simulink model "qpsk_tx"  (R2018a)
settings: Solver=VariableStepAuto  StartTime=0.0  StopTime=1e-6  RelTol=1e-3
libraries: simulink x2, commdigbbndpm3 x1, commfilt2 x1
settings Model: Creator=alist  LastModifiedBy=alist

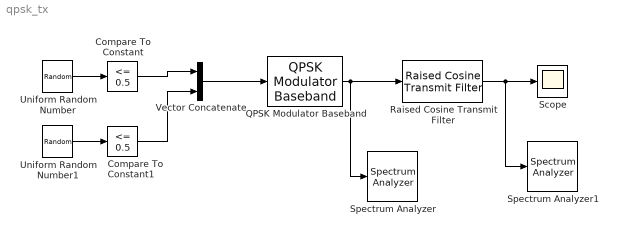
== system qpsk_tx ==
  Compare To Constant : simulink/Logic and Bit Operations/Compare To Constant  relop=<=  const=0.5  OutDataTypeStr=boolean
  Compare To Constant1 : simulink/Logic and Bit Operations/Compare To Constant  relop=<=  const=0.5  OutDataTypeStr=boolean
  QPSK Modulator Baseband : commdigbbndpm3/QPSK Modulator Baseband  InType=Bit  Enc=Gray  Ph=pi/4  outDtype=double  outWordLen=16  outUDDataType=sfix(16)  outFracLenMode=Best precision  outFracLen=15  outDataTypeStr=double  outLastDataTypeStr=double
  Raised Cosine Transmit Filter : commfilt2/Raised Cosine Transmit Filter  filtType=Square root  R=0.2  filtSpan=10  N=8  filterGain=1  InputProcessing=Columns as channels (frame based)  RateOptions=Enforce single-rate processing  framing=Mute  checkCoeff=off  variableName=rcTxFilt  checkGain=Normalized  sampMode=Mute  saveAsFlag=0  currentFiltSpan=10  D=(10)/2  launchFVT=on  roundingMode=Floor  overflowMode=off  coeffDataTypeStr=Inherit: Same word length as input  coeffMin=[]  coeffMax=[]  coeffLastDataTypeStr=Inherit: Same word length as input  outputDataTypeStr=Inherit: Same as accumulator  outputMin=[]  outputMax=[]  outputLastDataTypeStr=Inherit: Same as accumulator
  Scope : Scope
  Spectrum Analyzer : SpectrumAnalyzer
  Spectrum Analyzer1 : SpectrumAnalyzer
  Uniform Random Number : UniformRandomNumber  Minimum=0  SampleTime=50e-9
  Uniform Random Number1 : UniformRandomNumber  Minimum=0  Seed=1  SampleTime=50e-9
  Vector Concatenate : Concatenate
  wires:
  Uniform Random Number/1 -> Compare To Constant/1
  Uniform Random Number1/1 -> Compare To Constant1/1
  Compare To Constant/1 -> Vector Concatenate/1
  Compare To Constant1/1 -> Vector Concatenate/2
  Vector Concatenate/1 -> QPSK Modulator Baseband/1
  QPSK Modulator Baseband/1 -> Raised Cosine Transmit Filter/1, Spectrum Analyzer/1
  Raised Cosine Transmit Filter/1 -> Scope/1, Spectrum Analyzer1/1
